simulink model "power_48pulsegtoconverter"  (Simulink 6.0)
settings: Solver=FixedStepDiscrete  SolverMode=SingleTasking  StartTime=0.0  StopTime=0.05  RelTol=1e-3
libraries: powerlib x17, powerlib_extras x1
(part 1 of 2)
settings Model: Creator=hyp01  LastModifiedBy=batserve  ExtModeTrigMode=oneshot  ExtModeArmWhenConnect=off  ExtModeAutoUpdateStatusClock=off
settings DataIOCC: LimitDataPoints=off  SaveOutput=off  SaveTime=off  SignalLoggingName=sigsOut
settings OptimizationCC: BlockReduction=off  BooleanDataType=off
settings DebuggingCC: CheckExecutionContextPreStartOutputMsg=on  CheckExecutionContextRuntimeOutputMsg=on  SolverPrmCheckMsg=none
settings HardwareCC: TargetUnknown=on

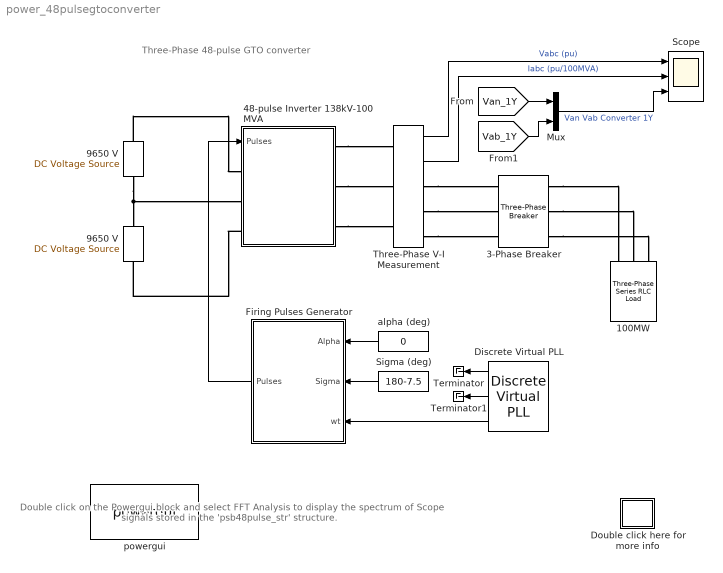
== system power_48pulsegtoconverter ==
  note: Three-Phase 48-pulse GTO converter
  note: Double click on the Powergui block and
      | select FFT Analysis to display the
      | spectrum of Scope  signals stored in the
      | 'psb48pulse_str' structure.
  100MW : powerlib/Elements/Three-Phase Series RLC Load  Orientation=down  PhysicalDomain=powersysdomain  SubClassName=unknown  LeftPortType=p1  RightPortType=p1  LConnTagsString=A|B|C  Configuration=Y (grounded)  NominalVoltage=138e3  NominalFrequency=60  ActivePower=100e6  InductivePower=0  CapacitivePower=0  Measurements=None
  3-Phase Breaker : powerlib/Elements/Three-Phase Breaker  InitialState=open  SwitchA=on  SwitchB=on  SwitchC=on  SwitchTimes=[0.025]  External=off  BreakerResistance=0.001  SnubberResistance=1e6  SnubberCapacitance=inf  Measurements=None
      settings: AttributesFormatString=\n
  48-pulse Inverter 138kV-100 MVA : Subsystem
  "9650 V " : powerlib/Electrical Sources/DC Voltage Source  Description=source block  Orientation=up  Amplitude=9650  Measurements=None
      settings: AttributesFormatString=\n
  "9650 V  " : powerlib/Electrical Sources/DC Voltage Source  Description=source block  Orientation=up  Amplitude=9650  Measurements=None
      settings: AttributesFormatString=\n
  Discrete Virtual PLL : powerlib_extras/Discrete  Control Blocks/Discrete Virtual PLL  Orientation=left  Freq=60  Phase=0  Ts=5e-6
  Double click here for more info : Subsystem
      mask Display: disp('?')
  Firing Pulses Generator : Subsystem  Orientation=left
  Mux : Mux  Inputs=2
  Scope : Scope  NumInputPorts=3
      settings: TimeRange=0.05  YMin=-2~-1~-20000  YMax=2~1~20000  SaveName=psb48pulse_str  SampleInput=on  SampleTime=-1
  Sigma (deg) : Constant  Orientation=left  Value=180-7.5
  Terminator : Terminator
  Terminator1 : Terminator
  Three-Phase V-I Measurement : powerlib/Measurements/Three-Phase V-I Measurement  VoltageMeasurement=phase-to-ground  SetLabelV=off  LabelV=V1  Vpu=on  Vbase=138e3  CurrentMeasurement=yes  SetLabelI=off  LabelI=I1  Ipu=on  Pbase=100e6  OutputType=Magnitude  PhasorSimulation=off  PSBequivalent=0
  alpha (deg) : Constant  Orientation=left  Value=0  VectorParams1D=off
  powergui : powerlib/powergui  Priority=2  Frange=logspace(0,3,50)  Ylog=off  Xlog=off  save=off  variable=ZData  structure=psb48pulse_str  ZoomFFT=on  StartTime=0.025-1/60  cycles=1  DisplayStyle=off  fundamental=60  FreqAxis=on  MaxFrequency=4000  frequencyindice=1  frequencyindicesteady=1  RmsSteady=1  display=off  Ts=5e-6  methode=off  frequency=60  echomessages=on
  wires:
  Sigma (deg)/1 -> Firing Pulses Generator/2(Sigma)
  Discrete Virtual PLL/1 -> Terminator/1
  Discrete Virtual PLL/2 -> Terminator1/1
  Firing Pulses Generator/1(Pulses) -> 48-pulse Inverter 138kV-100 MVA/1(Pulses)
  Discrete Virtual PLL/3 -> Firing Pulses Generator/3(wt)
  alpha (deg)/1 -> Firing Pulses Generator/1(Alpha)
  [Van_1Y] -> Mux/1
  [Vab_1Y] -> Mux/2
  Three-Phase V-I Measurement/1 -> Scope/1  "Vabc (pu)"
  Mux/1 -> Scope/3  "Van Vab Converter 1Y"
  Three-Phase V-I Measurement/2 -> Scope/2  "Iabc (pu/100MVA)"
  connections:
  3-Phase Breaker/RConn1 -- 100MW/LConn1
  3-Phase Breaker/RConn2 -- 100MW/LConn2
  3-Phase Breaker/RConn3 -- 100MW/LConn3
  "9650 V  "/LConn1 -- "9650 V "/RConn1 -- 48-pulse Inverter 138kV-100 MVA/LConn2
  48-pulse Inverter 138kV-100 MVA/RConn1 -- Three-Phase V-I Measurement/LConn1
  48-pulse Inverter 138kV-100 MVA/RConn2 -- Three-Phase V-I Measurement/LConn2
  48-pulse Inverter 138kV-100 MVA/RConn3 -- Three-Phase V-I Measurement/LConn3
  Three-Phase V-I Measurement/RConn1 -- 3-Phase Breaker/LConn1
  Three-Phase V-I Measurement/RConn2 -- 3-Phase Breaker/LConn2
  Three-Phase V-I Measurement/RConn3 -- 3-Phase Breaker/LConn3
  "9650 V  "/RConn1 -- 48-pulse Inverter 138kV-100 MVA/LConn1
  48-pulse Inverter 138kV-100 MVA/LConn3 -- "9650 V "/LConn1

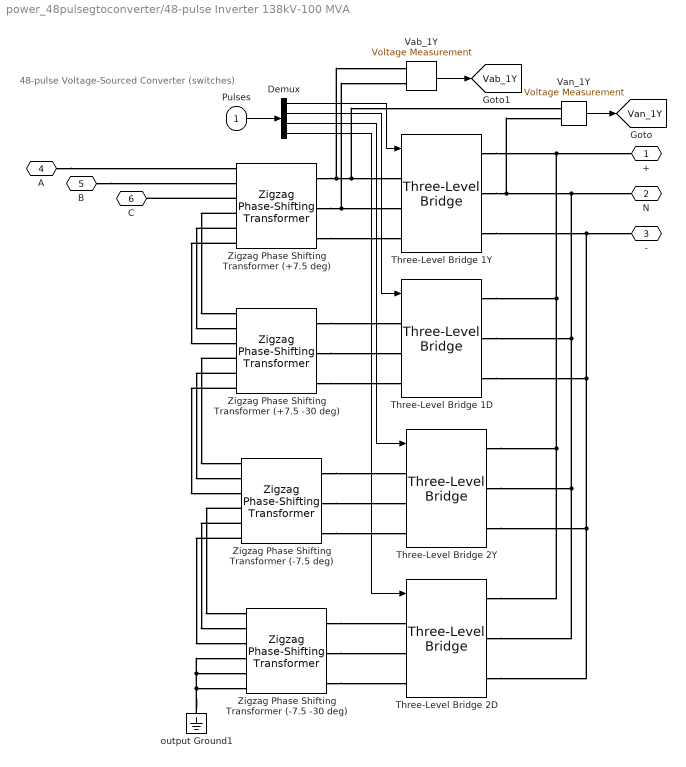
== system power_48pulsegtoconverter/48-pulse Inverter 138kV-100 MVA ==
  note: 48-pulse Voltage-Sourced Converter
      | (switches)
  Pulses : Inport  Port=1  PortDimensions=48  LatchInput=off
  Demux : Demux  Outputs=[12 12 12 12]
  Three-Level Bridge 1D : powerlib/Power Electronics/Three-Level Bridge  Arms=3  SnubberResistance=1e6  SbubberCapacitance=inf  Device=Ideal Switches  Ron=1e-4  ForwardVoltages="[  0  0  ]"  Measurements=None
  Three-Level Bridge 1Y : powerlib/Power Electronics/Three-Level Bridge  Arms=3  SnubberResistance=1e6  SbubberCapacitance=inf  Device=Ideal Switches  Ron=1e-4  ForwardVoltages="[  0  0  ]"  Measurements=None
  Three-Level Bridge 2D : powerlib/Power Electronics/Three-Level Bridge  Arms=3  SnubberResistance=1e6  SbubberCapacitance=inf  Device=Ideal Switches  Ron=1e-4  ForwardVoltages="[  0  0  ]"  Measurements=None
  Three-Level Bridge 2Y : powerlib/Power Electronics/Three-Level Bridge  Arms=3  SnubberResistance=1e6  SbubberCapacitance=inf  Device=Ideal Switches  Ron=1e-4  ForwardVoltages="[  0  0  ]"  Measurements=None
  Vab_1Y : powerlib/Measurements/Voltage Measurement  Tag=PoWeRsYsTeMmEaSuReMeNt  PhasorSimulation=off  OutputType=Magnitude  PSBequivalent=0
  Van_1Y : powerlib/Measurements/Voltage Measurement  Tag=PoWeRsYsTeMmEaSuReMeNt  PhasorSimulation=off  OutputType=Magnitude  PSBequivalent=0
  Zigzag Phase Shifting Transformer (+7.5 -30 deg) : powerlib/Elements/Zigzag Phase-Shifting Transformer  NominalPower=[ 25e6 60]  PrimaryVoltage=138e3/4  SecondaryVoltage="[ 15e3  +7.5]"  SecondaryConnection=Delta D1(-30 deg.)  Winding1=[ 0.00125 0.05 ]  Winding2=[ 0.00125 0.05 ]  Winding3=[ 0.00125 0.05 ]  SetSaturation=off  RmLm=[ 500 500 ]  Rm=500  Saturation="[ 0,0  ;  0.005,1.2  ;  1.0,1.4 ]"  Measurements=Fluxes and magnetization currents (Imag)  InitialFluxes=[0,0,0]
      settings: AttributesFormatString=\n
  Zigzag Phase Shifting Transformer (+7.5 deg) : powerlib/Elements/Zigzag Phase-Shifting Transformer  NominalPower=[ 25e6 60]  PrimaryVoltage=138e3/4  SecondaryVoltage="[ 15e3  +7.5]"  SecondaryConnection=Y  Winding1=[ 0.00125 0.05 ]  Winding2=[ 0.00125 0.05 ]  Winding3=[ 0.00125 0.05 ]  SetSaturation=off  RmLm=[ 500 500 ]  Rm=500  Saturation="[ 0,0  ;  0.005,1.2  ;  1.0,1.4 ]"  Measurements=Fluxes and excitation currents (Imag + IRm)  InitialFluxes=[0,0,0]
      settings: AttributesFormatString=\n
  Zigzag Phase Shifting Transformer (-7.5 -30 deg) : powerlib/Elements/Zigzag Phase-Shifting Transformer  NominalPower=[ 25e6 60]  PrimaryVoltage=138e3/4  SecondaryVoltage="[ 15e3  -7.5]"  SecondaryConnection=Delta D1(-30 deg.)  Winding1=[ 0.00125 0.05 ]  Winding2=[ 0.00125 0.05 ]  Winding3=[ 0.00125 0.05 ]  SetSaturation=off  RmLm=[ 500 500 ]  Rm=500  Saturation="[ 0,0  ;  0.005,1.2  ;  1.0,1.4 ]"  Measurements=None  InitialFluxes=[0,0,0]
      settings: AttributesFormatString=\n
  Zigzag Phase Shifting Transformer (-7.5 deg) : powerlib/Elements/Zigzag Phase-Shifting Transformer  NominalPower=[ 25e6 60]  PrimaryVoltage=138e3/4  SecondaryVoltage="[ 15e3  -7.5]"  SecondaryConnection=Y  Winding1=[ 0.00125 0.05 ]  Winding2=[ 0.00125 0.05 ]  Winding3=[ 0.00125 0.05 ]  SetSaturation=off  RmLm=[ 500 500 ]  Rm=500  Saturation="[ 0,0  ;  0.005,1.2  ;  1.0,1.4 ]"  Measurements=None  InitialFluxes=[0,0,0]
      settings: AttributesFormatString=\n
  output Ground1 : powerlib/Elements/Ground  Orientation=down  PhysicalDomain=powersysdomain  SubClassName=unknown  LeftPortType=p1  RightPortType=p1  LConnTagsString=a
  + : PMIOPort  Orientation=left  Port=1  Side=Left
  N : PMIOPort  Orientation=left  Port=2  Side=Left
  - : PMIOPort  Orientation=left  Port=3  Side=Left
  A : PMIOPort  Port=4  Side=Right
  B : PMIOPort  Port=5  Side=Right
  C : PMIOPort  Port=6  Side=Right
  tag scope: Vab_1Y=global, Van_1Y=global
  wires:
  Pulses/1 -> Demux/1
  Van_1Y/1 -> [Van_1Y]
  Vab_1Y/1 -> [Vab_1Y]
  Demux/1 -> Three-Level Bridge 1Y/1
  Demux/2 -> Three-Level Bridge 1D/1
  Demux/3 -> Three-Level Bridge 2Y/1
  Demux/4 -> Three-Level Bridge 2D/1
  connections:
  output Ground1/LConn1 -- Zigzag Phase Shifting Transformer (-7.5 -30 deg)/LConn5 -- Zigzag Phase Shifting Transformer (-7.5 -30 deg)/LConn4 -- Zigzag Phase Shifting Transformer (-7.5 -30 deg)/LConn6
  Zigzag Phase Shifting Transformer (+7.5 -30 deg)/RConn1 -- Three-Level Bridge 1D/LConn1
  Zigzag Phase Shifting Transformer (+7.5 -30 deg)/RConn2 -- Three-Level Bridge 1D/LConn2
  Zigzag Phase Shifting Transformer (+7.5 -30 deg)/RConn3 -- Three-Level Bridge 1D/LConn3
  Zigzag Phase Shifting Transformer (-7.5 deg)/RConn1 -- Three-Level Bridge 2Y/LConn1
  Zigzag Phase Shifting Transformer (-7.5 deg)/RConn2 -- Three-Level Bridge 2Y/LConn2
  Zigzag Phase Shifting Transformer (-7.5 deg)/RConn3 -- Three-Level Bridge 2Y/LConn3
  Zigzag Phase Shifting Transformer (-7.5 -30 deg)/RConn1 -- Three-Level Bridge 2D/LConn1
  Zigzag Phase Shifting Transformer (-7.5 -30 deg)/RConn2 -- Three-Level Bridge 2D/LConn2
  Zigzag Phase Shifting Transformer (-7.5 -30 deg)/RConn3 -- Three-Level Bridge 2D/LConn3
  A/RConn1 -- Zigzag Phase Shifting Transformer (+7.5 deg)/LConn1
  B/RConn1 -- Zigzag Phase Shifting Transformer (+7.5 deg)/LConn2
  Zigzag Phase Shifting Transformer (+7.5 deg)/LConn3 -- C/RConn1
  Zigzag Phase Shifting Transformer (+7.5 deg)/RConn2 -- Three-Level Bridge 1Y/LConn2 -- Vab_1Y/LConn2
  Zigzag Phase Shifting Transformer (+7.5 deg)/RConn1 -- Vab_1Y/LConn1 -- Three-Level Bridge 1Y/LConn1 -- Van_1Y/LConn1
  Zigzag Phase Shifting Transformer (+7.5 deg)/RConn3 -- Three-Level Bridge 1Y/LConn3
  Zigzag Phase Shifting Transformer (+7.5 deg)/LConn4 -- Zigzag Phase Shifting Transformer (+7.5 -30 deg)/LConn1
  Zigzag Phase Shifting Transformer (+7.5 deg)/LConn5 -- Zigzag Phase Shifting Transformer (+7.5 -30 deg)/LConn2
  Zigzag Phase Shifting Transformer (+7.5 deg)/LConn6 -- Zigzag Phase Shifting Transformer (+7.5 -30 deg)/LConn3
  Zigzag Phase Shifting Transformer (+7.5 -30 deg)/LConn4 -- Zigzag Phase Shifting Transformer (-7.5 deg)/LConn1
  Zigzag Phase Shifting Transformer (+7.5 -30 deg)/LConn5 -- Zigzag Phase Shifting Transformer (-7.5 deg)/LConn2
  Zigzag Phase Shifting Transformer (+7.5 -30 deg)/LConn6 -- Zigzag Phase Shifting Transformer (-7.5 deg)/LConn3
  Zigzag Phase Shifting Transformer (-7.5 deg)/LConn5 -- Zigzag Phase Shifting Transformer (-7.5 -30 deg)/LConn2
  Three-Level Bridge 1Y/RConn2 -- N/RConn1 -- Three-Level Bridge 1D/RConn2 -- Three-Level Bridge 2D/RConn2 -- Three-Level Bridge 2Y/RConn2 -- Van_1Y/LConn2
  Three-Level Bridge 2D/RConn1 -- Three-Level Bridge 2Y/RConn1 -- Three-Level Bridge 1Y/RConn1 -- +/RConn1 -- Three-Level Bridge 1D/RConn1
  Three-Level Bridge 2D/RConn3 -- Three-Level Bridge 2Y/RConn3 -- Three-Level Bridge 1Y/RConn3 -- -/RConn1 -- Three-Level Bridge 1D/RConn3
  Zigzag Phase Shifting Transformer (-7.5 deg)/LConn4 -- Zigzag Phase Shifting Transformer (-7.5 -30 deg)/LConn1
  Zigzag Phase Shifting Transformer (-7.5 deg)/LConn6 -- Zigzag Phase Shifting Transformer (-7.5 -30 deg)/LConn3

== system power_48pulsegtoconverter/Double click here for more info ==
  note: Run the simulation and observe the following  waveforms on the Scope block:
      |
      | Voltages generated by the inverter (trace 1), load currents (trace 2), phase-neutral voltage and phase-phase voltage of one of  the four inverters (1Y) superimposed on trace 3.
      | When the inverter is operating at no load, you can observe the three 48-step voltage waveform. When the load is switched on the voltage becomes smoother because harmonics
      | are filtered by the transformer leakage reactances.
      |
      | Once the  simulation is completed, open the Powergui and select  "FFT Analysis" to display the 0-4000 Hz frequency spectrum of signals saved
      | in the two "psb48pulse_str" structure. Select signal labeled 'Vabc (pu)'. The FFT will be performed on a 1-cycle window of phase A voltage starting at t = 0.025-1/60 s
      | (inverter operating at no load). Click on Display and observe the frequency spectrum.
      |
      | The fundamental component of  Voltage (in pu) as well as THD  are displayed above the spectrum window.
      | Notice that the first significant harmonics are 47th and 49th (approx. 2%). Notice also that 23rd and 25th are reduced below 0.3%.
      | In order to appreciate the efficiency of harmonic neutralization, you can also observe the frequency spectrum of phase-phase voltage generated by each individual inverter.
      | Select input labeled  "Van Vab Converter 1Y" and signal number 2 and click on Display. Observe that THD in the 0 - 4000 Hz frequency range is 25%.
      |
      | You can also run another simulation by specifying different values of sigma at the input of the pulse generator.
      | You can verify that, in order to cancel a particular harmonic n in the phase-phase voltage of each individual converter, the Sigma value (in degrees) is given by:
      |
      |      Sigma=180*(1 - 1/n)
      |
      | Verify also that choosing Sigma = 180 degrees is equivalent to using 2-level converters and that voltage waveform is degraded to 24 pulses.
  note: In this example, ideal switches and zig-zag phase shifting  transformers are used to build a GTO-type 100 MVA, 138 kV voltage source inverter.
      | This type of converter is used in high-power (up to 200 MVA) Flexible AC Transmission Systems (FACTS) which are used to control power flow on transmission grids.
      | It can be used, for example, to build a model of shunt or series static compensator (STATCOM or SSSC) or, using two such converters, a combination of shunt and series
      | devices known as Unified Power Flow Controller (UPFC).
      |
      | The inverter described in this example is a harmonic neutralized, 48-pulse GTO converter described in reference. It consists of four 3-phase, 3-level inverters and
      | four phase-shifting transformers. Open the "48-pulse inverter" subsystem. Notice that the DC bus (Vdc = +/-9650 V) is connected to the four 3-phase inverters.The four voltages
      | generated by the inverters are applied to secondary windings of four zig-zag phase-shifting transformers connected in Wye (Y) or Delta (D). The four transformer primary windings are
      | connected in series and the converter pulse patterns are phase shifted so that the four voltage fundamental components sum in phase on the primary side.
      |
      | Each 3-level inverter generates three square-wave voltages which can be +Vdc, 0, -Vdc. The duration of the +Vdc or -Vdc level (Sigma) can be adjusted  between 0 and 180
      | degrees from the Sigma input of the Firing Pulse Generator block.
      | Each inverter uses a Three-Level Bridge block where specified power electronic devices are Ideal Switches. In this model each leg of the inverter uses 3 ideal switches
      | to obtain the 3 voltage levels (+Vdc, 0, - Vdc).  This simple model simulates the behavior of a physical inverter where each leg consists of 4 GTOs, 4 antiparallel diodes and
      | 2 neutral clamping diodes. Despite this simplified switch arrangement, the model still requires 4 pulses per arm as in the physical model.
      | The pulse pattern sent to each leg of a 3-phase inverter is described inside the Firing Pulse Generator.
      |
      | You can also select GTO/Diodes pairs instead of Ideal Switches as power electronic devices. It would allow you to specify forward voltage drops for GTOs and diodes
      | and to observe currents flowing in GTOs and diodes  by means of the Multimeter block.
      |
      | The phase shifts produced by the secondary delta connections (-30 degrees) and by the primary zig-zag connections (+7.5 degrees for transformers 1Y and 1D, and -7.5 degrees
      | for transformers 2Y and 2D) allows to neutralize harmonics up to 45th harmonic, as explained below:
      |
      | The 30-degree phase-shift between the Y and D secondaries cancels harmonics 5+12n (5, 17, 29, 41, ...) and 7+12n (7, 19, 31, 43, ...). In addition, the 15-degree phase shift between
      | the two groups of transformers (1Y and 1D leading by 7.5 degrees, 2Y and 2D lagging by +7.5 degrees) allows cancellation of harmonics 11+24n (11, 35, ...) and 13+24n (13, 37, ...).
      | Considering that all 3n the harmonics are not transmitted by the Y and D secondaries, the first harmonic which are not cancelled by the transformers are 23rd, 25th, 47th and 49th.
      | By choosing an appropriate conduction angle for the 3-level inverters (sigma = 180 - 7.5 = 172.5 degrees), the 23rd and 25th can be minimized. The first significant harmonics are
      | therefore the 47th and 49th. This type of inverter generates an almost sinusoidal waveform consisting of  48-steps.
      |
      | The inverter is operated in open loop at constant DC voltage. During the first three cycles the inverter operates at no load. Then, at t = 0.05 s, a 100 MVA resistive load
      | is connected at the 138-kV terminals.
  note: This demonstration illustrates use of 3-level converters and zig-zag phase-shifting
      | transformers in a 48-pulse square-wave GTO converter.  It also demonstrates harmonic
      | analysis using the Powergui/FFT tool.
  note: Circuit Description
  note: Demonstration
  note: P. Giroux and G. Sybille (Hydro-Quebec)
  note: Reference:
  note: Narain G. Hingorani and Laszlo Gyuyi, "Understanding FACTS", IEEE Press , 2000

== system power_48pulsegtoconverter/Firing Pulses Generator ==
  Alpha : Inport  Port=1  PortDimensions=1  LatchInput=off
  Sigma : Inport  Port=2  PortDimensions=1  LatchInput=off
  wt : Inport  Port=3  PortDimensions=1  LatchInput=off
  Bridge 1D : Subsystem
  "Bridge 1Y " : Subsystem
  Bridge 2D : Subsystem
  Bridge 2Y : Subsystem
  Constant : Constant  Value=[0 -30 -15 -45]*pi/180
  Deg->Rad : Gain  Gain=pi/180  SaturateOnIntegerOverflow=on
  "Deg->Rad " : Gain  Gain=pi/180  SaturateOnIntegerOverflow=on
  Demux : Demux
  Mux : Mux  Inputs=[12 12 12 12]
  Sum : Sum  SaturateOnIntegerOverflow=on  InputSameDT=on
  Pulses : Outport
  wires:
  Alpha/1 -> Deg->Rad/1
  Constant/1 -> Sum/2
  "Bridge 1Y "/1(Pulses) -> Mux/1
  Mux/1 -> Pulses/1
  Demux/1 -> "Bridge 1Y "/1(wt)
  Sigma/1 -> "Deg->Rad "/1
  Demux/2 -> Bridge 1D/1(wt)
  Demux/3 -> Bridge 2Y/1(wt)
  Demux/4 -> Bridge 2D/1(wt)
  Deg->Rad/1 -> "Bridge 1Y "/2(Alpha), Bridge 2Y/2(Alpha), Bridge 2D/2(Alpha), Bridge 1D/2(Alpha)
  "Deg->Rad "/1 -> "Bridge 1Y "/3(Sigma), Bridge 1D/3(Sigma), Bridge 2Y/3(Sigma), Bridge 2D/3(Sigma)
  Bridge 1D/1(Pulses) -> Mux/2
  Bridge 2Y/1(Pulses) -> Mux/3
  Bridge 2D/1(Pulses) -> Mux/4
  wt/1 -> Sum/1
  Sum/1 -> Demux/1

== system power_48pulsegtoconverter/Firing Pulses Generator/Bridge 1D ==
  wt : Inport  Port=1  PortDimensions=1  LatchInput=off
  Alpha : Inport  Port=2  PortDimensions=1  LatchInput=off
  Sigma : Inport  Port=3  PortDimensions=1  LatchInput=off
  Constant : Constant  Value=-2*pi/3
  Constant1 : Constant  Value=2*pi/3
  Mux1 : Mux  Inputs=[4 4 4]
  Phase A : Subsystem
  Phase B : Subsystem
  Phase C : Subsystem
  Sum : Sum  SaturateOnIntegerOverflow=on  InputSameDT=on
  Sum1 : Sum  SaturateOnIntegerOverflow=on  InputSameDT=on
  Sum2 : Sum  SaturateOnIntegerOverflow=on  InputSameDT=on
  Pulses : Outport
  wires:
  Constant1/1 -> Sum1/2
  Sigma/1 -> Phase A/2(sigma), Phase C/2(sigma), Phase B/2(sigma)
  Alpha/1 -> Sum2/2
  wt/1 -> Sum2/1
  Sum2/1 -> Phase A/1(wt), Sum/1, Sum1/1
  Mux1/1 -> Pulses/1
  Phase A/1(Pulses) -> Mux1/1
  Constant/1 -> Sum/2
  Sum/1 -> Phase B/1(wt)
  Sum1/1 -> Phase C/1(wt)
  Phase B/1(Pulses) -> Mux1/2
  Phase C/1(Pulses) -> Mux1/3

== system power_48pulsegtoconverter/Firing Pulses Generator/Bridge 1Y  ==
  wt : Inport  Port=1  PortDimensions=1  LatchInput=off
  Alpha : Inport  Port=2  PortDimensions=1  LatchInput=off
  Sigma : Inport  Port=3  PortDimensions=1  LatchInput=off
  Constant : Constant  Value=-2*pi/3
  Constant1 : Constant  Value=2*pi/3
  Mux1 : Mux  Inputs=[4 4 4]
  Phase A : Subsystem
  Phase B : Subsystem
  Phase C : Subsystem
  Sum : Sum  SaturateOnIntegerOverflow=on  InputSameDT=on
  Sum1 : Sum  SaturateOnIntegerOverflow=on  InputSameDT=on
  Sum2 : Sum  SaturateOnIntegerOverflow=on  InputSameDT=on
  Pulses : Outport
  wires:
  Phase C/1(Pulses) -> Mux1/3
  Phase B/1(Pulses) -> Mux1/2
  Sum1/1 -> Phase C/1(wt)
  Sum/1 -> Phase B/1(wt)
  Constant/1 -> Sum/2
  Phase A/1(Pulses) -> Mux1/1
  Mux1/1 -> Pulses/1
  Sum2/1 -> Sum1/1, Sum/1, Phase A/1(wt)
  wt/1 -> Sum2/1
  Alpha/1 -> Sum2/2
  Sigma/1 -> Phase B/2(sigma), Phase C/2(sigma), Phase A/2(sigma)
  Constant1/1 -> Sum1/2

== system power_48pulsegtoconverter/Firing Pulses Generator/Bridge 2D ==
  wt : Inport  Port=1  PortDimensions=1  LatchInput=off
  Alpha : Inport  Port=2  PortDimensions=1  LatchInput=off
  Sigma : Inport  Port=3  PortDimensions=1  LatchInput=off
  Constant : Constant  Value=-2*pi/3
  Constant1 : Constant  Value=2*pi/3
  Mux1 : Mux  Inputs=[4 4 4]
  Phase A : Subsystem
  Phase B : Subsystem
  Phase C : Subsystem
  Sum : Sum  SaturateOnIntegerOverflow=on  InputSameDT=on
  Sum1 : Sum  SaturateOnIntegerOverflow=on  InputSameDT=on
  Sum2 : Sum  SaturateOnIntegerOverflow=on  InputSameDT=on
  Pulses : Outport
  wires:
  Constant1/1 -> Sum1/2
  Sigma/1 -> Phase A/2(sigma), Phase C/2(sigma), Phase B/2(sigma)
  Alpha/1 -> Sum2/2
  wt/1 -> Sum2/1
  Sum2/1 -> Phase A/1(wt), Sum/1, Sum1/1
  Mux1/1 -> Pulses/1
  Phase A/1(Pulses) -> Mux1/1
  Constant/1 -> Sum/2
  Sum/1 -> Phase B/1(wt)
  Sum1/1 -> Phase C/1(wt)
  Phase B/1(Pulses) -> Mux1/2
  Phase C/1(Pulses) -> Mux1/3

== system power_48pulsegtoconverter/Firing Pulses Generator/Bridge 2Y ==
  wt : Inport  Port=1  PortDimensions=1  LatchInput=off
  Alpha : Inport  Port=2  PortDimensions=1  LatchInput=off
  Sigma : Inport  Port=3  PortDimensions=1  LatchInput=off
  Constant : Constant  Value=-2*pi/3
  Constant1 : Constant  Value=2*pi/3
  Mux1 : Mux  Inputs=[4 4 4]
  Phase A : Subsystem
  Phase B : Subsystem
  Phase C : Subsystem
  Sum : Sum  SaturateOnIntegerOverflow=on  InputSameDT=on
  Sum1 : Sum  SaturateOnIntegerOverflow=on  InputSameDT=on
  Sum2 : Sum  SaturateOnIntegerOverflow=on  InputSameDT=on
  Pulses : Outport
  wires:
  Phase C/1(Pulses) -> Mux1/3
  Phase B/1(Pulses) -> Mux1/2
  Sum1/1 -> Phase C/1(wt)
  Sum/1 -> Phase B/1(wt)
  Constant/1 -> Sum/2
  Phase A/1(Pulses) -> Mux1/1
  Mux1/1 -> Pulses/1
  Sum2/1 -> Sum1/1, Sum/1, Phase A/1(wt)
  wt/1 -> Sum2/1
  Alpha/1 -> Sum2/2
  Sigma/1 -> Phase B/2(sigma), Phase C/2(sigma), Phase A/2(sigma)
  Constant1/1 -> Sum1/2

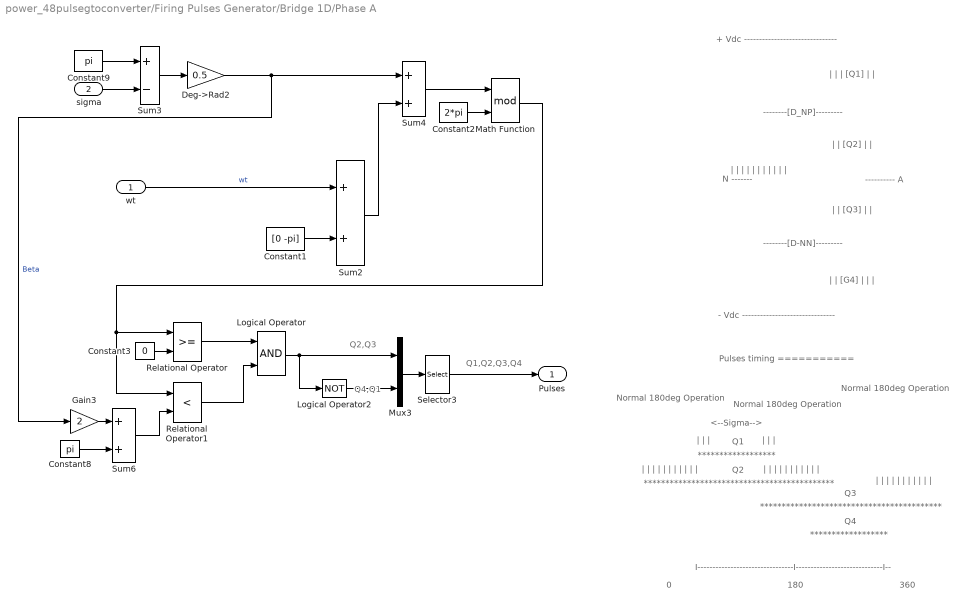
== system power_48pulsegtoconverter/Firing Pulses Generator/Bridge 1D/Phase A ==
  note: <--Sigma-->
  note: |
      | |
      | |
  note: |
      | |
      | |
  note: Q4
  note: Q3
  note: Q2
  note: Q1
  note: ******************************************
  note: ********************************************
  note: ******************
  note: ******************
  note: 360
  note: 180
  note: 0
  note: I--------------------------------I-----------------------------I--
  note: Normal 180deg
      | Operation
  note: Normal 180deg
      | Operation
  note: Normal 180deg
      | Operation
  note: Pulses timing
      | ===========
  note: |
      | |
      | |
      | |
      | |
      | |
      | |
      | |
      | |
      | |
      | |
  note: |
      | |
      | |
      | |
      | |
      | |
      | |
      | |
      | |
      | |
      | |
  note: |
      | |
      | |
      | |
      | |
      | |
      | |
      | |
      | |
      | |
      | |
  note: Q1,Q2,Q3,Q4
  note: Q2,Q3
  note: Q4,Q1
  note: + Vdc -------------------------------
  note: - Vdc -------------------------------
  note: N -------
  note: |
      | |
      | |
      | |
      | |
      | |
      | |
      | |
      | |
      | |
      | |
  note: ---------- A
  note: --------[D-NN]---------
  note: --------[D_NP]---------
  note: |
      | |
      | [G4]
      | |
      | |
      | |
  note: |
      | |
      | [Q3]
      | |
      | |
  note: |
      | |
      | [Q2]
      | |
      | |
  note: |
      | |
      | |
      | [Q1]
      | |
      | |
  wt : Inport  Port=1  PortDimensions=1  LatchInput=off
  sigma : Inport  Port=2  PortDimensions=1  LatchInput=off
  Constant1 : Constant  Value=[0 -pi]
  Constant2 : Constant  Value=2*pi
  Constant3 : Constant  Value=0
  Constant8 : Constant  Value=pi
  Constant9 : Constant  Value=pi
  Deg->Rad2 : Gain  Gain=0.5  SaturateOnIntegerOverflow=on
  Gain3 : Gain  Gain=2  SaturateOnIntegerOverflow=on
  Logical Operator : Logic
  Logical Operator2 : Logic  Operator=NOT
  Math Function : Math  Operator=mod  SaturateOnIntegerOverflow=on
  Mux3 : Mux  Inputs=[2 2]
  Relational Operator : RelationalOperator  ZeroCross=off  InputSameDT=on
  Relational Operator1 : RelationalOperator  Operator=<  ZeroCross=off  InputSameDT=on
  Selector3 : Selector  Elements=[4 1 2 3]  InputPortWidth=4
  Sum2 : Sum  SaturateOnIntegerOverflow=on  InputSameDT=on
  Sum3 : Sum  Inputs=+-  SaturateOnIntegerOverflow=on  InputSameDT=on
  Sum4 : Sum  SaturateOnIntegerOverflow=on  InputSameDT=on
  Sum6 : Sum  SaturateOnIntegerOverflow=on  InputSameDT=on
  Pulses : Outport
  wires:
  Constant2/1 -> Math Function/2
  wt/1 -> Sum2/1  "wt"
  Math Function/1 -> Relational Operator/1, Relational Operator1/1
  Gain3/1 -> Sum6/1
  Selector3/1 -> Pulses/1
  Mux3/1 -> Selector3/1
  Logical Operator2/1 -> Mux3/2
  Logical Operator/1 -> Mux3/1, Logical Operator2/1
  Sum4/1 -> Math Function/1
  Sum2/1 -> Sum4/2
  Sum6/1 -> Relational Operator1/2
  Constant8/1 -> Sum6/2
  Deg->Rad2/1 -> Gain3/1, Sum4/1  "Beta"
  Sum3/1 -> Deg->Rad2/1
  sigma/1 -> Sum3/2
  Constant9/1 -> Sum3/1
  Relational Operator1/1 -> Logical Operator/2
  Relational Operator/1 -> Logical Operator/1
  Constant3/1 -> Relational Operator/2
  Constant1/1 -> Sum2/2

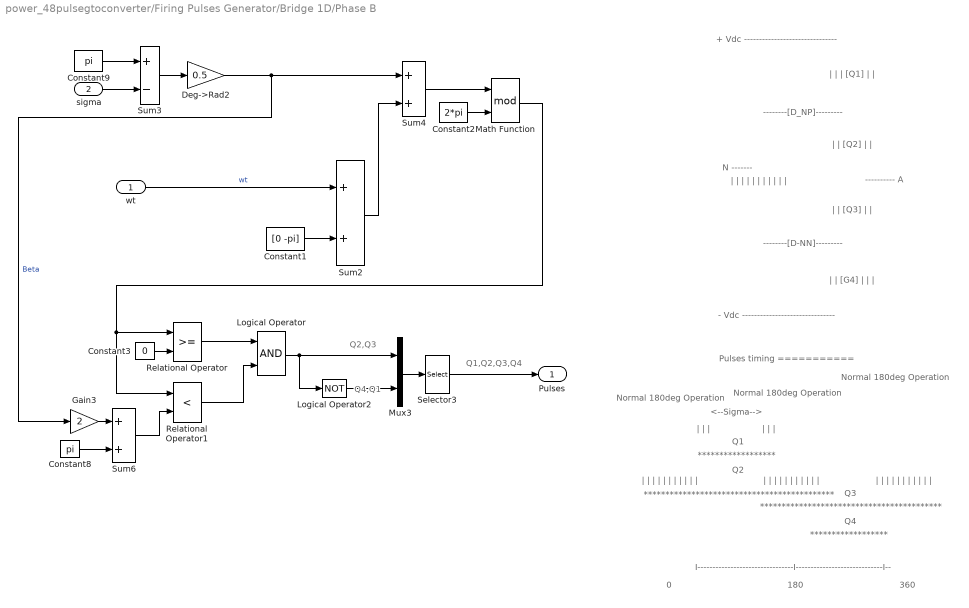
== system power_48pulsegtoconverter/Firing Pulses Generator/Bridge 1D/Phase B ==
  note: |
      | |
      | |
      | [Q1]
      | |
      | |
  note: |
      | |
      | [Q2]
      | |
      | |
  note: |
      | |
      | [Q3]
      | |
      | |
  note: |
      | |
      | [G4]
      | |
      | |
      | |
  note: --------[D_NP]---------
  note: --------[D-NN]---------
  note: ---------- A
  note: |
      | |
      | |
      | |
      | |
      | |
      | |
      | |
      | |
      | |
      | |
  note: N -------
  note: - Vdc -------------------------------
  note: + Vdc -------------------------------
  note: Q4,Q1
  note: Q2,Q3
  note: Q1,Q2,Q3,Q4
  note: |
      | |
      | |
      | |
      | |
      | |
      | |
      | |
      | |
      | |
      | |
  note: |
      | |
      | |
      | |
      | |
      | |
      | |
      | |
      | |
      | |
      | |
  note: |
      | |
      | |
      | |
      | |
      | |
      | |
      | |
      | |
      | |
      | |
  note: Pulses timing
      | ===========
  note: Normal 180deg
      | Operation
  note: Normal 180deg
      | Operation
  note: Normal 180deg
      | Operation
  note: I--------------------------------I-----------------------------I--
  note: 0
  note: 180
  note: 360
  note: ******************
  note: ******************
  note: ********************************************
  note: ******************************************
  note: Q1
  note: Q2
  note: Q3
  note: Q4
  note: |
      | |
      | |
  note: |
      | |
      | |
  note: <--Sigma-->
  wt : Inport  Port=1  PortDimensions=1  LatchInput=off
  sigma : Inport  Port=2  PortDimensions=1  LatchInput=off
  Constant1 : Constant  Value=[0 -pi]
  Constant2 : Constant  Value=2*pi
  Constant3 : Constant  Value=0
  Constant8 : Constant  Value=pi
  Constant9 : Constant  Value=pi
  Deg->Rad2 : Gain  Gain=0.5  SaturateOnIntegerOverflow=on
  Gain3 : Gain  Gain=2  SaturateOnIntegerOverflow=on
  Logical Operator : Logic
  Logical Operator2 : Logic  Operator=NOT
  Math Function : Math  Operator=mod  SaturateOnIntegerOverflow=on
  Mux3 : Mux  Inputs=[2 2]
  Relational Operator : RelationalOperator  ZeroCross=off  InputSameDT=on
  Relational Operator1 : RelationalOperator  Operator=<  ZeroCross=off  InputSameDT=on
  Selector3 : Selector  Elements=[4 1 2 3]  InputPortWidth=4
  Sum2 : Sum  SaturateOnIntegerOverflow=on  InputSameDT=on
  Sum3 : Sum  Inputs=+-  SaturateOnIntegerOverflow=on  InputSameDT=on
  Sum4 : Sum  SaturateOnIntegerOverflow=on  InputSameDT=on
  Sum6 : Sum  SaturateOnIntegerOverflow=on  InputSameDT=on
  Pulses : Outport
  wires:
  Constant1/1 -> Sum2/2
  Constant3/1 -> Relational Operator/2
  Relational Operator/1 -> Logical Operator/1
  Relational Operator1/1 -> Logical Operator/2
  Constant9/1 -> Sum3/1
  sigma/1 -> Sum3/2
  Sum3/1 -> Deg->Rad2/1
  Deg->Rad2/1 -> Sum4/1, Gain3/1  "Beta"
  Constant8/1 -> Sum6/2
  Sum6/1 -> Relational Operator1/2
  Sum2/1 -> Sum4/2
  Sum4/1 -> Math Function/1
  Logical Operator/1 -> Logical Operator2/1, Mux3/1
  Logical Operator2/1 -> Mux3/2
  Mux3/1 -> Selector3/1
  Selector3/1 -> Pulses/1
  Gain3/1 -> Sum6/1
  Math Function/1 -> Relational Operator1/1, Relational Operator/1
  wt/1 -> Sum2/1  "wt"
  Constant2/1 -> Math Function/2

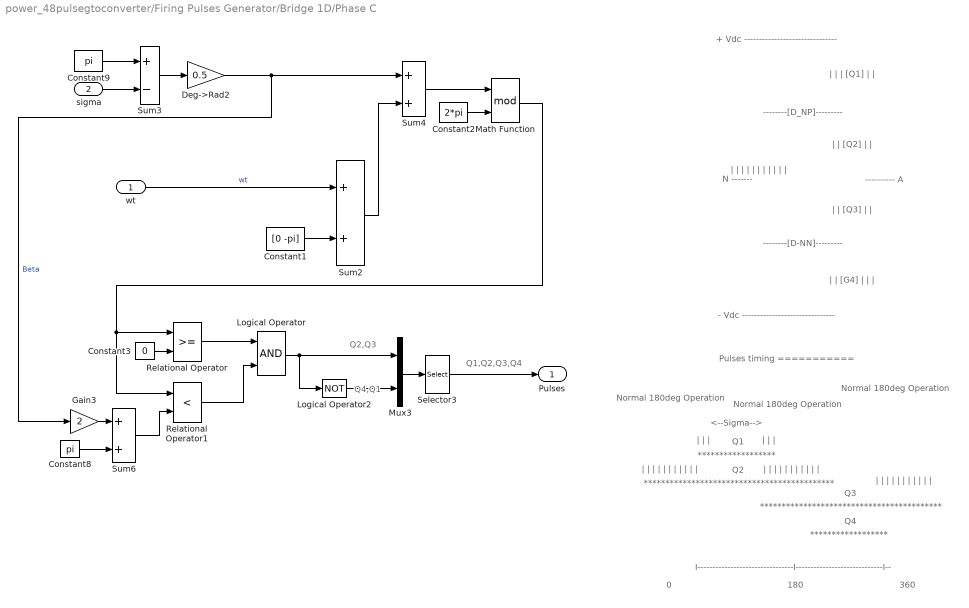
== system power_48pulsegtoconverter/Firing Pulses Generator/Bridge 1D/Phase C ==
  note: <--Sigma-->
  note: |
      | |
      | |
  note: |
      | |
      | |
  note: Q4
  note: Q3
  note: Q2
  note: Q1
  note: ******************************************
  note: ********************************************
  note: ******************
  note: ******************
  note: 360
  note: 180
  note: 0
  note: I--------------------------------I-----------------------------I--
  note: Normal 180deg
      | Operation
  note: Normal 180deg
      | Operation
  note: Normal 180deg
      | Operation
  note: Pulses timing
      | ===========
  note: |
      | |
      | |
      | |
      | |
      | |
      | |
      | |
      | |
      | |
      | |
  note: |
      | |
      | |
      | |
      | |
      | |
      | |
      | |
      | |
      | |
      | |
  note: |
      | |
      | |
      | |
      | |
      | |
      | |
      | |
      | |
      | |
      | |
  note: Q1,Q2,Q3,Q4
  note: Q2,Q3
  note: Q4,Q1
  note: + Vdc -------------------------------
  note: - Vdc -------------------------------
  note: N -------
  note: |
      | |
      | |
      | |
      | |
      | |
      | |
      | |
      | |
      | |
      | |
  note: ---------- A
  note: --------[D-NN]---------
  note: --------[D_NP]---------
  note: |
      | |
      | [G4]
      | |
      | |
      | |
  note: |
      | |
      | [Q3]
      | |
      | |
  note: |
      | |
      | [Q2]
      | |
      | |
  note: |
      | |
      | |
      | [Q1]
      | |
      | |
  wt : Inport  Port=1  PortDimensions=1  LatchInput=off
  sigma : Inport  Port=2  PortDimensions=1  LatchInput=off
  Constant1 : Constant  Value=[0 -pi]
  Constant2 : Constant  Value=2*pi
  Constant3 : Constant  Value=0
  Constant8 : Constant  Value=pi
  Constant9 : Constant  Value=pi
  Deg->Rad2 : Gain  Gain=0.5  SaturateOnIntegerOverflow=on
  Gain3 : Gain  Gain=2  SaturateOnIntegerOverflow=on
  Logical Operator : Logic
  Logical Operator2 : Logic  Operator=NOT
  Math Function : Math  Operator=mod  SaturateOnIntegerOverflow=on
  Mux3 : Mux  Inputs=[2 2]
  Relational Operator : RelationalOperator  ZeroCross=off  InputSameDT=on
  Relational Operator1 : RelationalOperator  Operator=<  ZeroCross=off  InputSameDT=on
  Selector3 : Selector  Elements=[4 1 2 3]  InputPortWidth=4
  Sum2 : Sum  SaturateOnIntegerOverflow=on  InputSameDT=on
  Sum3 : Sum  Inputs=+-  SaturateOnIntegerOverflow=on  InputSameDT=on
  Sum4 : Sum  SaturateOnIntegerOverflow=on  InputSameDT=on
  Sum6 : Sum  SaturateOnIntegerOverflow=on  InputSameDT=on
  Pulses : Outport
  wires:
  Constant2/1 -> Math Function/2
  wt/1 -> Sum2/1  "wt"
  Math Function/1 -> Relational Operator/1, Relational Operator1/1
  Gain3/1 -> Sum6/1
  Selector3/1 -> Pulses/1
  Mux3/1 -> Selector3/1
  Logical Operator2/1 -> Mux3/2
  Logical Operator/1 -> Mux3/1, Logical Operator2/1
  Sum4/1 -> Math Function/1
  Sum2/1 -> Sum4/2
  Sum6/1 -> Relational Operator1/2
  Constant8/1 -> Sum6/2
  Deg->Rad2/1 -> Gain3/1, Sum4/1  "Beta"
  Sum3/1 -> Deg->Rad2/1
  sigma/1 -> Sum3/2
  Constant9/1 -> Sum3/1
  Relational Operator1/1 -> Logical Operator/2
  Relational Operator/1 -> Logical Operator/1
  Constant3/1 -> Relational Operator/2
  Constant1/1 -> Sum2/2

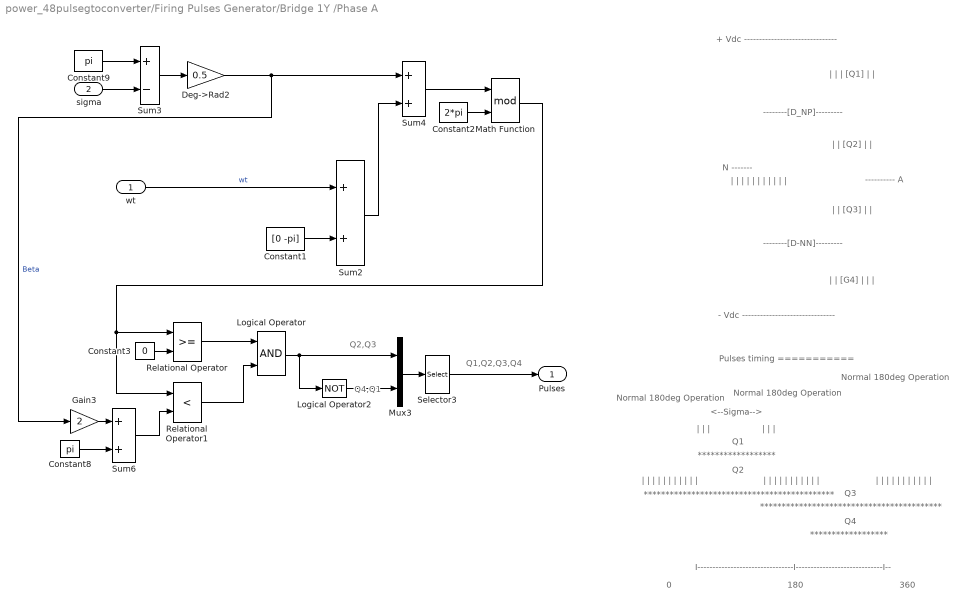
== system power_48pulsegtoconverter/Firing Pulses Generator/Bridge 1Y /Phase A ==
  note: |
      | |
      | |
      | [Q1]
      | |
      | |
  note: |
      | |
      | [Q2]
      | |
      | |
  note: |
      | |
      | [Q3]
      | |
      | |
  note: |
      | |
      | [G4]
      | |
      | |
      | |
  note: --------[D_NP]---------
  note: --------[D-NN]---------
  note: ---------- A
  note: |
      | |
      | |
      | |
      | |
      | |
      | |
      | |
      | |
      | |
      | |
  note: N -------
  note: - Vdc -------------------------------
  note: + Vdc -------------------------------
  note: Q4,Q1
  note: Q2,Q3
  note: Q1,Q2,Q3,Q4
  note: |
      | |
      | |
      | |
      | |
      | |
      | |
      | |
      | |
      | |
      | |
  note: |
      | |
      | |
      | |
      | |
      | |
      | |
      | |
      | |
      | |
      | |
  note: |
      | |
      | |
      | |
      | |
      | |
      | |
      | |
      | |
      | |
      | |
  note: Pulses timing
      | ===========
  note: Normal 180deg
      | Operation
  note: Normal 180deg
      | Operation
  note: Normal 180deg
      | Operation
  note: I--------------------------------I-----------------------------I--
  note: 0
  note: 180
  note: 360
  note: ******************
  note: ******************
  note: ********************************************
  note: ******************************************
  note: Q1
  note: Q2
  note: Q3
  note: Q4
  note: |
      | |
      | |
  note: |
      | |
      | |
  note: <--Sigma-->
  wt : Inport  Port=1  PortDimensions=1  LatchInput=off
  sigma : Inport  Port=2  PortDimensions=1  LatchInput=off
  Constant1 : Constant  Value=[0 -pi]
  Constant2 : Constant  Value=2*pi
  Constant3 : Constant  Value=0
  Constant8 : Constant  Value=pi
  Constant9 : Constant  Value=pi
  Deg->Rad2 : Gain  Gain=0.5  SaturateOnIntegerOverflow=on
  Gain3 : Gain  Gain=2  SaturateOnIntegerOverflow=on
  Logical Operator : Logic
  Logical Operator2 : Logic  Operator=NOT
  Math Function : Math  Operator=mod  SaturateOnIntegerOverflow=on
  Mux3 : Mux  Inputs=[2 2]
  Relational Operator : RelationalOperator  ZeroCross=off  InputSameDT=on
  Relational Operator1 : RelationalOperator  Operator=<  ZeroCross=off  InputSameDT=on
  Selector3 : Selector  Elements=[4 1 2 3]  InputPortWidth=4
  Sum2 : Sum  SaturateOnIntegerOverflow=on  InputSameDT=on
  Sum3 : Sum  Inputs=+-  SaturateOnIntegerOverflow=on  InputSameDT=on
  Sum4 : Sum  SaturateOnIntegerOverflow=on  InputSameDT=on
  Sum6 : Sum  SaturateOnIntegerOverflow=on  InputSameDT=on
  Pulses : Outport
  wires:
  Constant1/1 -> Sum2/2
  Constant3/1 -> Relational Operator/2
  Relational Operator/1 -> Logical Operator/1
  Relational Operator1/1 -> Logical Operator/2
  Constant9/1 -> Sum3/1
  sigma/1 -> Sum3/2
  Sum3/1 -> Deg->Rad2/1
  Deg->Rad2/1 -> Sum4/1, Gain3/1  "Beta"
  Constant8/1 -> Sum6/2
  Sum6/1 -> Relational Operator1/2
  Sum2/1 -> Sum4/2
  Sum4/1 -> Math Function/1
  Logical Operator/1 -> Logical Operator2/1, Mux3/1
  Logical Operator2/1 -> Mux3/2
  Mux3/1 -> Selector3/1
  Selector3/1 -> Pulses/1
  Gain3/1 -> Sum6/1
  Math Function/1 -> Relational Operator1/1, Relational Operator/1
  wt/1 -> Sum2/1  "wt"
  Constant2/1 -> Math Function/2

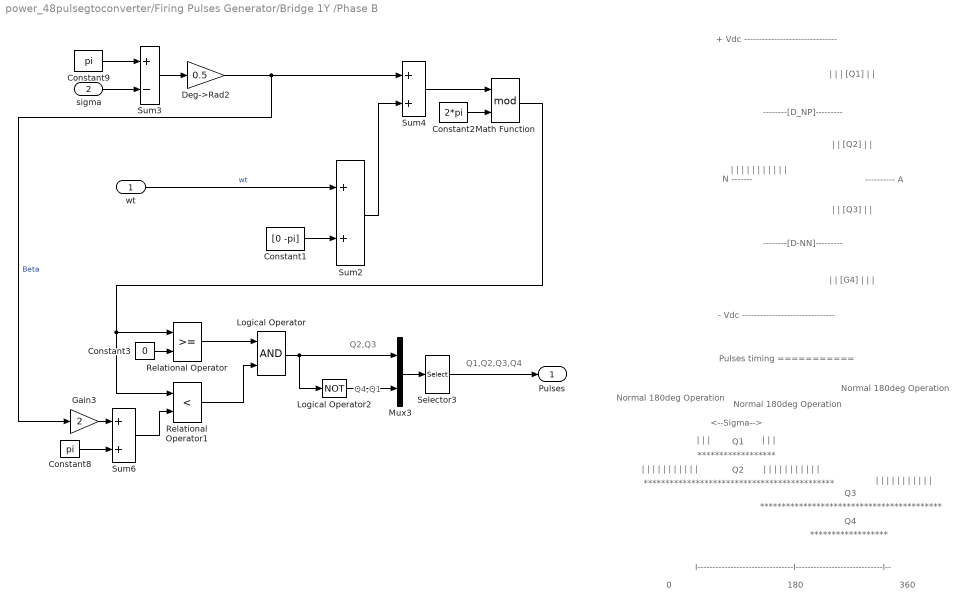
== system power_48pulsegtoconverter/Firing Pulses Generator/Bridge 1Y /Phase B ==
  note: <--Sigma-->
  note: |
      | |
      | |
  note: |
      | |
      | |
  note: Q4
  note: Q3
  note: Q2
  note: Q1
  note: ******************************************
  note: ********************************************
  note: ******************
  note: ******************
  note: 360
  note: 180
  note: 0
  note: I--------------------------------I-----------------------------I--
  note: Normal 180deg
      | Operation
  note: Normal 180deg
      | Operation
  note: Normal 180deg
      | Operation
  note: Pulses timing
      | ===========
  note: |
      | |
      | |
      | |
      | |
      | |
      | |
      | |
      | |
      | |
      | |
  note: |
      | |
      | |
      | |
      | |
      | |
      | |
      | |
      | |
      | |
      | |
  note: |
      | |
      | |
      | |
      | |
      | |
      | |
      | |
      | |
      | |
      | |
  note: Q1,Q2,Q3,Q4
  note: Q2,Q3
  note: Q4,Q1
  note: + Vdc -------------------------------
  note: - Vdc -------------------------------
  note: N -------
  note: |
      | |
      | |
      | |
      | |
      | |
      | |
      | |
      | |
      | |
      | |
  note: ---------- A
  note: --------[D-NN]---------
  note: --------[D_NP]---------
  note: |
      | |
      | [G4]
      | |
      | |
      | |
  note: |
      | |
      | [Q3]
      | |
      | |
  note: |
      | |
      | [Q2]
      | |
      | |
  note: |
      | |
      | |
      | [Q1]
      | |
      | |
  wt : Inport  Port=1  PortDimensions=1  LatchInput=off
  sigma : Inport  Port=2  PortDimensions=1  LatchInput=off
  Constant1 : Constant  Value=[0 -pi]
  Constant2 : Constant  Value=2*pi
  Constant3 : Constant  Value=0
  Constant8 : Constant  Value=pi
  Constant9 : Constant  Value=pi
  Deg->Rad2 : Gain  Gain=0.5  SaturateOnIntegerOverflow=on
  Gain3 : Gain  Gain=2  SaturateOnIntegerOverflow=on
  Logical Operator : Logic
  Logical Operator2 : Logic  Operator=NOT
  Math Function : Math  Operator=mod  SaturateOnIntegerOverflow=on
  Mux3 : Mux  Inputs=[2 2]
  Relational Operator : RelationalOperator  ZeroCross=off  InputSameDT=on
  Relational Operator1 : RelationalOperator  Operator=<  ZeroCross=off  InputSameDT=on
  Selector3 : Selector  Elements=[4 1 2 3]  InputPortWidth=4
  Sum2 : Sum  SaturateOnIntegerOverflow=on  InputSameDT=on
  Sum3 : Sum  Inputs=+-  SaturateOnIntegerOverflow=on  InputSameDT=on
  Sum4 : Sum  SaturateOnIntegerOverflow=on  InputSameDT=on
  Sum6 : Sum  SaturateOnIntegerOverflow=on  InputSameDT=on
  Pulses : Outport
  wires:
  Constant2/1 -> Math Function/2
  wt/1 -> Sum2/1  "wt"
  Math Function/1 -> Relational Operator/1, Relational Operator1/1
  Gain3/1 -> Sum6/1
  Selector3/1 -> Pulses/1
  Mux3/1 -> Selector3/1
  Logical Operator2/1 -> Mux3/2
  Logical Operator/1 -> Mux3/1, Logical Operator2/1
  Sum4/1 -> Math Function/1
  Sum2/1 -> Sum4/2
  Sum6/1 -> Relational Operator1/2
  Constant8/1 -> Sum6/2
  Deg->Rad2/1 -> Gain3/1, Sum4/1  "Beta"
  Sum3/1 -> Deg->Rad2/1
  sigma/1 -> Sum3/2
  Constant9/1 -> Sum3/1
  Relational Operator1/1 -> Logical Operator/2
  Relational Operator/1 -> Logical Operator/1
  Constant3/1 -> Relational Operator/2
  Constant1/1 -> Sum2/2

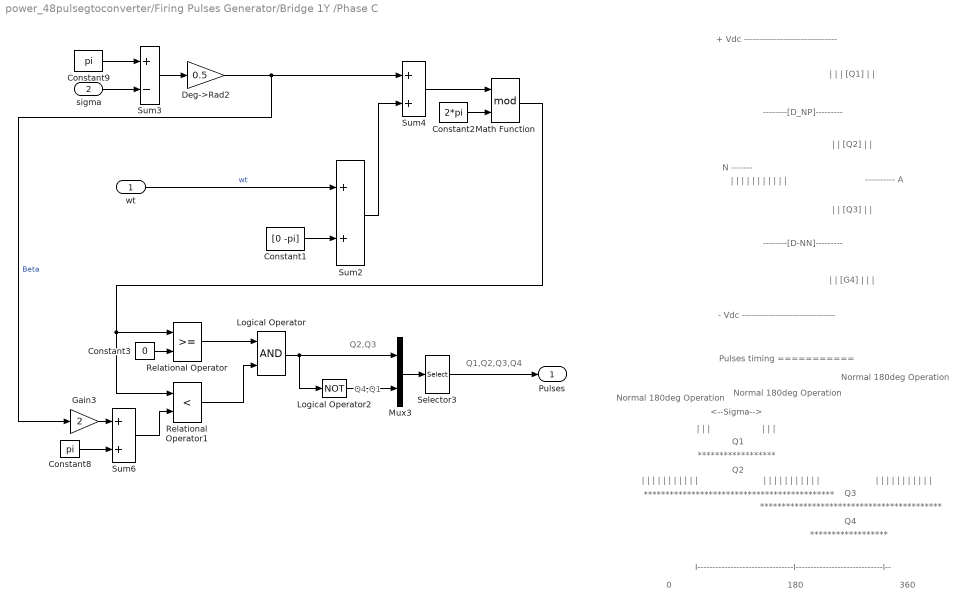
== system power_48pulsegtoconverter/Firing Pulses Generator/Bridge 1Y /Phase C ==
  note: |
      | |
      | |
      | [Q1]
      | |
      | |
  note: |
      | |
      | [Q2]
      | |
      | |
  note: |
      | |
      | [Q3]
      | |
      | |
  note: |
      | |
      | [G4]
      | |
      | |
      | |
  note: --------[D_NP]---------
  note: --------[D-NN]---------
  note: ---------- A
  note: |
      | |
      | |
      | |
      | |
      | |
      | |
      | |
      | |
      | |
      | |
  note: N -------
  note: - Vdc -------------------------------
  note: + Vdc -------------------------------
  note: Q4,Q1
  note: Q2,Q3
  note: Q1,Q2,Q3,Q4
  note: |
      | |
      | |
      | |
      | |
      | |
      | |
      | |
      | |
      | |
      | |
  note: |
      | |
      | |
      | |
      | |
      | |
      | |
      | |
      | |
      | |
      | |
  note: |
      | |
      | |
      | |
      | |
      | |
      | |
      | |
      | |
      | |
      | |
  note: Pulses timing
      | ===========
  note: Normal 180deg
      | Operation
  note: Normal 180deg
      | Operation
  note: Normal 180deg
      | Operation
  note: I--------------------------------I-----------------------------I--
  note: 0
  note: 180
  note: 360
  note: ******************
  note: ******************
  note: ********************************************
  note: ******************************************
  note: Q1
  note: Q2
  note: Q3
  note: Q4
  note: |
      | |
      | |
  note: |
      | |
      | |
  note: <--Sigma-->
  wt : Inport  Port=1  PortDimensions=1  LatchInput=off
  sigma : Inport  Port=2  PortDimensions=1  LatchInput=off
  Constant1 : Constant  Value=[0 -pi]
  Constant2 : Constant  Value=2*pi
  Constant3 : Constant  Value=0
  Constant8 : Constant  Value=pi
  Constant9 : Constant  Value=pi
  Deg->Rad2 : Gain  Gain=0.5  SaturateOnIntegerOverflow=on
  Gain3 : Gain  Gain=2  SaturateOnIntegerOverflow=on
  Logical Operator : Logic
  Logical Operator2 : Logic  Operator=NOT
  Math Function : Math  Operator=mod  SaturateOnIntegerOverflow=on
  Mux3 : Mux  Inputs=[2 2]
  Relational Operator : RelationalOperator  ZeroCross=off  InputSameDT=on
  Relational Operator1 : RelationalOperator  Operator=<  ZeroCross=off  InputSameDT=on
  Selector3 : Selector  Elements=[4 1 2 3]  InputPortWidth=4
  Sum2 : Sum  SaturateOnIntegerOverflow=on  InputSameDT=on
  Sum3 : Sum  Inputs=+-  SaturateOnIntegerOverflow=on  InputSameDT=on
  Sum4 : Sum  SaturateOnIntegerOverflow=on  InputSameDT=on
  Sum6 : Sum  SaturateOnIntegerOverflow=on  InputSameDT=on
  Pulses : Outport
  wires:
  Constant1/1 -> Sum2/2
  Constant3/1 -> Relational Operator/2
  Relational Operator/1 -> Logical Operator/1
  Relational Operator1/1 -> Logical Operator/2
  Constant9/1 -> Sum3/1
  sigma/1 -> Sum3/2
  Sum3/1 -> Deg->Rad2/1
  Deg->Rad2/1 -> Sum4/1, Gain3/1  "Beta"
  Constant8/1 -> Sum6/2
  Sum6/1 -> Relational Operator1/2
  Sum2/1 -> Sum4/2
  Sum4/1 -> Math Function/1
  Logical Operator/1 -> Logical Operator2/1, Mux3/1
  Logical Operator2/1 -> Mux3/2
  Mux3/1 -> Selector3/1
  Selector3/1 -> Pulses/1
  Gain3/1 -> Sum6/1
  Math Function/1 -> Relational Operator1/1, Relational Operator/1
  wt/1 -> Sum2/1  "wt"
  Constant2/1 -> Math Function/2

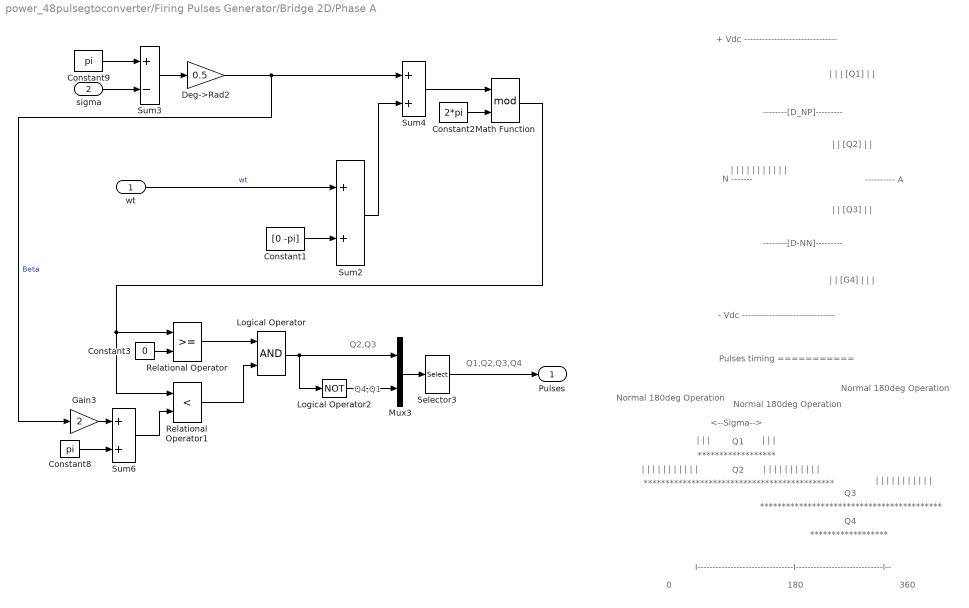
== system power_48pulsegtoconverter/Firing Pulses Generator/Bridge 2D/Phase A ==
  note: <--Sigma-->
  note: |
      | |
      | |
  note: |
      | |
      | |
  note: Q4
  note: Q3
  note: Q2
  note: Q1
  note: ******************************************
  note: ********************************************
  note: ******************
  note: ******************
  note: 360
  note: 180
  note: 0
  note: I--------------------------------I-----------------------------I--
  note: Normal 180deg
      | Operation
  note: Normal 180deg
      | Operation
  note: Normal 180deg
      | Operation
  note: Pulses timing
      | ===========
  note: |
      | |
      | |
      | |
      | |
      | |
      | |
      | |
      | |
      | |
      | |
  note: |
      | |
      | |
      | |
      | |
      | |
      | |
      | |
      | |
      | |
      | |
  note: |
      | |
      | |
      | |
      | |
      | |
      | |
      | |
      | |
      | |
      | |
  note: Q1,Q2,Q3,Q4
  note: Q2,Q3
  note: Q4,Q1
  note: + Vdc -------------------------------
  note: - Vdc -------------------------------
  note: N -------
  note: |
      | |
      | |
      | |
      | |
      | |
      | |
      | |
      | |
      | |
      | |
  note: ---------- A
  note: --------[D-NN]---------
  note: --------[D_NP]---------
  note: |
      | |
      | [G4]
      | |
      | |
      | |
  note: |
      | |
      | [Q3]
      | |
      | |
  note: |
      | |
      | [Q2]
      | |
      | |
  note: |
      | |
      | |
      | [Q1]
      | |
      | |
  wt : Inport  Port=1  PortDimensions=1  LatchInput=off
  sigma : Inport  Port=2  PortDimensions=1  LatchInput=off
  Constant1 : Constant  Value=[0 -pi]
  Constant2 : Constant  Value=2*pi
  Constant3 : Constant  Value=0
  Constant8 : Constant  Value=pi
  Constant9 : Constant  Value=pi
  Deg->Rad2 : Gain  Gain=0.5  SaturateOnIntegerOverflow=on
  Gain3 : Gain  Gain=2  SaturateOnIntegerOverflow=on
  Logical Operator : Logic
  Logical Operator2 : Logic  Operator=NOT
  Math Function : Math  Operator=mod  SaturateOnIntegerOverflow=on
  Mux3 : Mux  Inputs=[2 2]
  Relational Operator : RelationalOperator  ZeroCross=off  InputSameDT=on
  Relational Operator1 : RelationalOperator  Operator=<  ZeroCross=off  InputSameDT=on
  Selector3 : Selector  Elements=[4 1 2 3]  InputPortWidth=4
  Sum2 : Sum  SaturateOnIntegerOverflow=on  InputSameDT=on
  Sum3 : Sum  Inputs=+-  SaturateOnIntegerOverflow=on  InputSameDT=on
  Sum4 : Sum  SaturateOnIntegerOverflow=on  InputSameDT=on
  Sum6 : Sum  SaturateOnIntegerOverflow=on  InputSameDT=on
  Pulses : Outport
  wires:
  Constant2/1 -> Math Function/2
  wt/1 -> Sum2/1  "wt"
  Math Function/1 -> Relational Operator/1, Relational Operator1/1
  Gain3/1 -> Sum6/1
  Selector3/1 -> Pulses/1
  Mux3/1 -> Selector3/1
  Logical Operator2/1 -> Mux3/2
  Logical Operator/1 -> Mux3/1, Logical Operator2/1
  Sum4/1 -> Math Function/1
  Sum2/1 -> Sum4/2
  Sum6/1 -> Relational Operator1/2
  Constant8/1 -> Sum6/2
  Deg->Rad2/1 -> Gain3/1, Sum4/1  "Beta"
  Sum3/1 -> Deg->Rad2/1
  sigma/1 -> Sum3/2
  Constant9/1 -> Sum3/1
  Relational Operator1/1 -> Logical Operator/2
  Relational Operator/1 -> Logical Operator/1
  Constant3/1 -> Relational Operator/2
  Constant1/1 -> Sum2/2

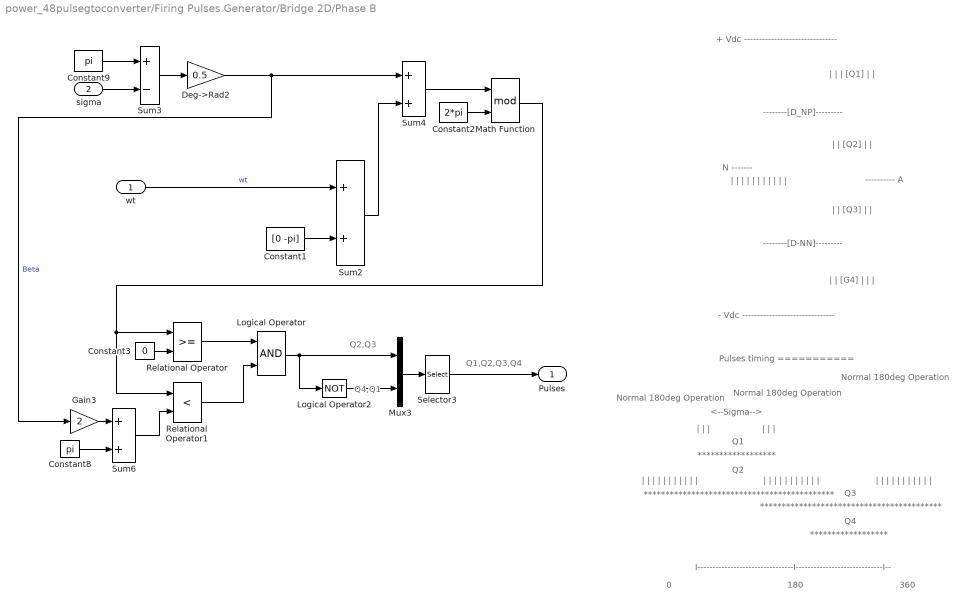
== system power_48pulsegtoconverter/Firing Pulses Generator/Bridge 2D/Phase B ==
  note: |
      | |
      | |
      | [Q1]
      | |
      | |
  note: |
      | |
      | [Q2]
      | |
      | |
  note: |
      | |
      | [Q3]
      | |
      | |
  note: |
      | |
      | [G4]
      | |
      | |
      | |
  note: --------[D_NP]---------
  note: --------[D-NN]---------
  note: ---------- A
  note: |
      | |
      | |
      | |
      | |
      | |
      | |
      | |
      | |
      | |
      | |
  note: N -------
  note: - Vdc -------------------------------
  note: + Vdc -------------------------------
  note: Q4,Q1
  note: Q2,Q3
  note: Q1,Q2,Q3,Q4
  note: |
      | |
      | |
      | |
      | |
      | |
      | |
      | |
      | |
      | |
      | |
  note: |
      | |
      | |
      | |
      | |
      | |
      | |
      | |
      | |
      | |
      | |
  note: |
      | |
      | |
      | |
      | |
      | |
      | |
      | |
      | |
      | |
      | |
  note: Pulses timing
      | ===========
  note: Normal 180deg
      | Operation
  note: Normal 180deg
      | Operation
  note: Normal 180deg
      | Operation
  note: I--------------------------------I-----------------------------I--
  note: 0
  note: 180
  note: 360
  note: ******************
  note: ******************
  note: ********************************************
  note: ******************************************
  note: Q1
  note: Q2
  note: Q3
  note: Q4
  note: |
      | |
      | |
  note: |
      | |
      | |
  note: <--Sigma-->
  wt : Inport  Port=1  PortDimensions=1  LatchInput=off
  sigma : Inport  Port=2  PortDimensions=1  LatchInput=off
  Constant1 : Constant  Value=[0 -pi]
  Constant2 : Constant  Value=2*pi
  Constant3 : Constant  Value=0
  Constant8 : Constant  Value=pi
  Constant9 : Constant  Value=pi
  Deg->Rad2 : Gain  Gain=0.5  SaturateOnIntegerOverflow=on
  Gain3 : Gain  Gain=2  SaturateOnIntegerOverflow=on
  Logical Operator : Logic
  Logical Operator2 : Logic  Operator=NOT
  Math Function : Math  Operator=mod  SaturateOnIntegerOverflow=on
  Mux3 : Mux  Inputs=[2 2]
  Relational Operator : RelationalOperator  ZeroCross=off  InputSameDT=on
  Relational Operator1 : RelationalOperator  Operator=<  ZeroCross=off  InputSameDT=on
  Selector3 : Selector  Elements=[4 1 2 3]  InputPortWidth=4
  Sum2 : Sum  SaturateOnIntegerOverflow=on  InputSameDT=on
  Sum3 : Sum  Inputs=+-  SaturateOnIntegerOverflow=on  InputSameDT=on
  Sum4 : Sum  SaturateOnIntegerOverflow=on  InputSameDT=on
  Sum6 : Sum  SaturateOnIntegerOverflow=on  InputSameDT=on
  Pulses : Outport
  wires:
  Constant1/1 -> Sum2/2
  Constant3/1 -> Relational Operator/2
  Relational Operator/1 -> Logical Operator/1
  Relational Operator1/1 -> Logical Operator/2
  Constant9/1 -> Sum3/1
  sigma/1 -> Sum3/2
  Sum3/1 -> Deg->Rad2/1
  Deg->Rad2/1 -> Sum4/1, Gain3/1  "Beta"
  Constant8/1 -> Sum6/2
  Sum6/1 -> Relational Operator1/2
  Sum2/1 -> Sum4/2
  Sum4/1 -> Math Function/1
  Logical Operator/1 -> Logical Operator2/1, Mux3/1
  Logical Operator2/1 -> Mux3/2
  Mux3/1 -> Selector3/1
  Selector3/1 -> Pulses/1
  Gain3/1 -> Sum6/1
  Math Function/1 -> Relational Operator1/1, Relational Operator/1
  wt/1 -> Sum2/1  "wt"
  Constant2/1 -> Math Function/2

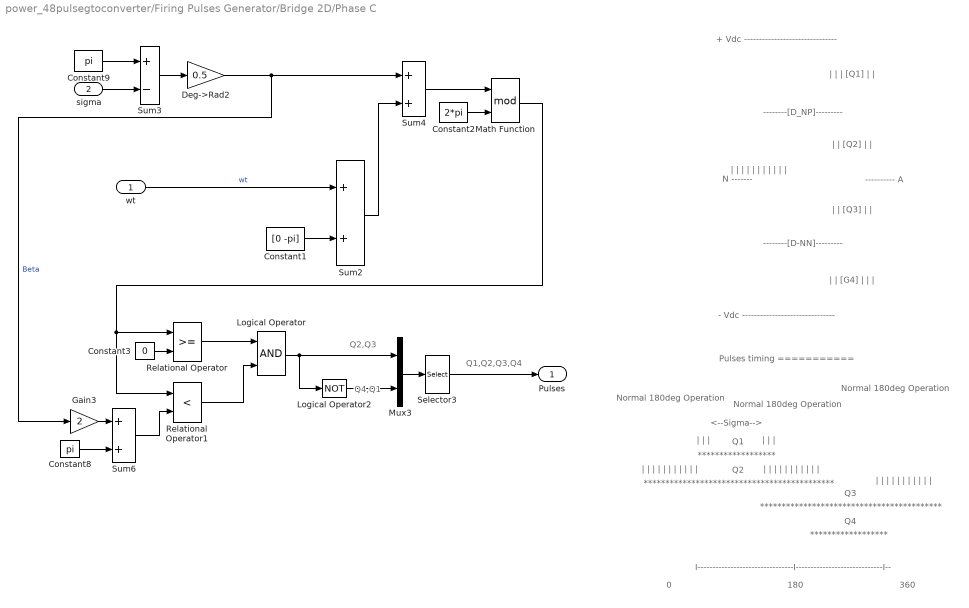
== system power_48pulsegtoconverter/Firing Pulses Generator/Bridge 2D/Phase C ==
  note: <--Sigma-->
  note: |
      | |
      | |
  note: |
      | |
      | |
  note: Q4
  note: Q3
  note: Q2
  note: Q1
  note: ******************************************
  note: ********************************************
  note: ******************
  note: ******************
  note: 360
  note: 180
  note: 0
  note: I--------------------------------I-----------------------------I--
  note: Normal 180deg
      | Operation
  note: Normal 180deg
      | Operation
  note: Normal 180deg
      | Operation
  note: Pulses timing
      | ===========
  note: |
      | |
      | |
      | |
      | |
      | |
      | |
      | |
      | |
      | |
      | |
  note: |
      | |
      | |
      | |
      | |
      | |
      | |
      | |
      | |
      | |
      | |
  note: |
      | |
      | |
      | |
      | |
      | |
      | |
      | |
      | |
      | |
      | |
  note: Q1,Q2,Q3,Q4
  note: Q2,Q3
  note: Q4,Q1
  note: + Vdc -------------------------------
  note: - Vdc -------------------------------
  note: N -------
  note: |
      | |
      | |
      | |
      | |
      | |
      | |
      | |
      | |
      | |
      | |
  note: ---------- A
  note: --------[D-NN]---------
  note: --------[D_NP]---------
  note: |
      | |
      | [G4]
      | |
      | |
      | |
  note: |
      | |
      | [Q3]
      | |
      | |
  note: |
      | |
      | [Q2]
      | |
      | |
  note: |
      | |
      | |
      | [Q1]
      | |
      | |
  wt : Inport  Port=1  PortDimensions=1  LatchInput=off
  sigma : Inport  Port=2  PortDimensions=1  LatchInput=off
  Constant1 : Constant  Value=[0 -pi]
  Constant2 : Constant  Value=2*pi
  Constant3 : Constant  Value=0
  Constant8 : Constant  Value=pi
  Constant9 : Constant  Value=pi
  Deg->Rad2 : Gain  Gain=0.5  SaturateOnIntegerOverflow=on
  Gain3 : Gain  Gain=2  SaturateOnIntegerOverflow=on
  Logical Operator : Logic
  Logical Operator2 : Logic  Operator=NOT
  Math Function : Math  Operator=mod  SaturateOnIntegerOverflow=on
  Mux3 : Mux  Inputs=[2 2]
  Relational Operator : RelationalOperator  ZeroCross=off  InputSameDT=on
  Relational Operator1 : RelationalOperator  Operator=<  ZeroCross=off  InputSameDT=on
  Selector3 : Selector  Elements=[4 1 2 3]  InputPortWidth=4
  Sum2 : Sum  SaturateOnIntegerOverflow=on  InputSameDT=on
  Sum3 : Sum  Inputs=+-  SaturateOnIntegerOverflow=on  InputSameDT=on
  Sum4 : Sum  SaturateOnIntegerOverflow=on  InputSameDT=on
  Sum6 : Sum  SaturateOnIntegerOverflow=on  InputSameDT=on
  Pulses : Outport
  wires:
  Constant2/1 -> Math Function/2
  wt/1 -> Sum2/1  "wt"
  Math Function/1 -> Relational Operator/1, Relational Operator1/1
  Gain3/1 -> Sum6/1
  Selector3/1 -> Pulses/1
  Mux3/1 -> Selector3/1
  Logical Operator2/1 -> Mux3/2
  Logical Operator/1 -> Mux3/1, Logical Operator2/1
  Sum4/1 -> Math Function/1
  Sum2/1 -> Sum4/2
  Sum6/1 -> Relational Operator1/2
  Constant8/1 -> Sum6/2
  Deg->Rad2/1 -> Gain3/1, Sum4/1  "Beta"
  Sum3/1 -> Deg->Rad2/1
  sigma/1 -> Sum3/2
  Constant9/1 -> Sum3/1
  Relational Operator1/1 -> Logical Operator/2
  Relational Operator/1 -> Logical Operator/1
  Constant3/1 -> Relational Operator/2
  Constant1/1 -> Sum2/2
